simulink subsystem "FMUEngine"  (R2024b)
settings: Solver=VariableStepAuto  StartTime=0.0  StopTime=10.0  RelTol=1e-3
undefined symbols (not defined in the file): Afr, BSFC, CrkAng, EngSpdOut, EngTrq, ExhManGasTemp, FuelFlw, FuelVolFlw, IntkPortFlw, NormAirChrg, PlntEngFuelSg
libraries: autolibhevctrlrcommon x1, autolibpowerinfoutils x1, autolibutils x1
settings Model: ModifiedByFormat=The MathWorks, Inc.  Creator=The MathWorks, Inc.  LastModifiedBy=The MathWorks, Inc.
settings OptimizationCC: ReuseModelBlockBuffer=off
settings DebuggingCC: SubsystemReferenceDiagnosticForUnitTest=warning
settings RTWCC: GPUComputeCapability=3.5

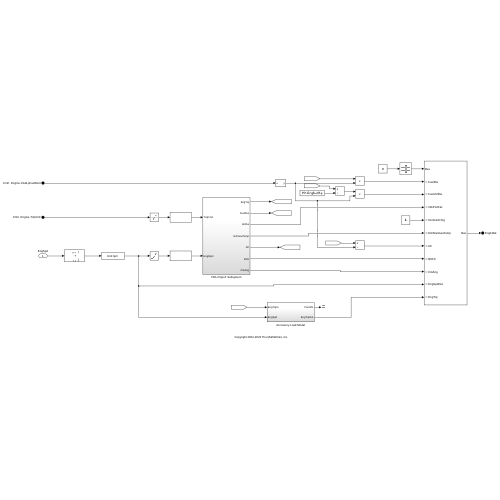
[thumbnail: Simulink's stored preview of the top-level diagram]
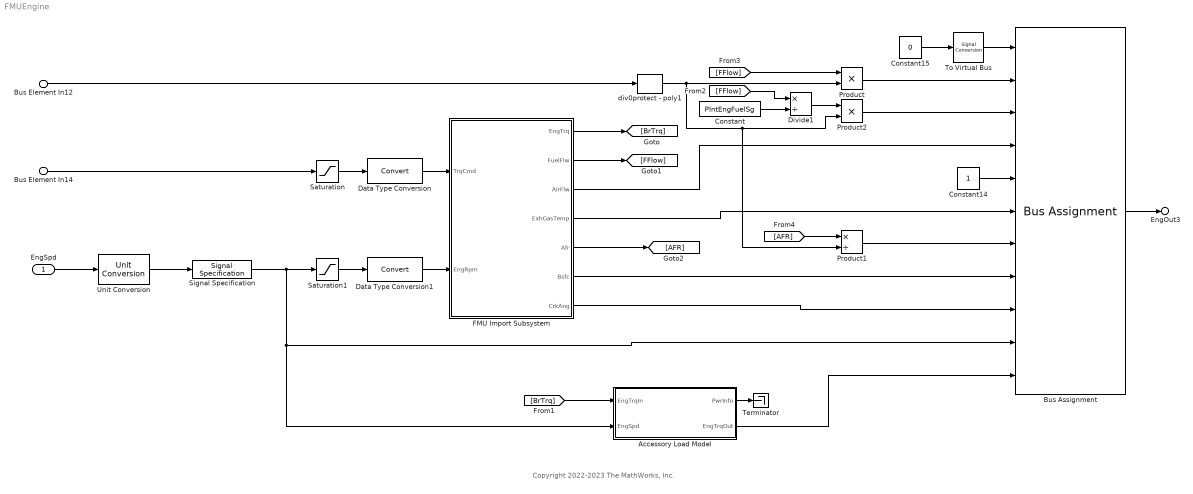
== system FMUEngine ==
  note: Copyright 2022-2023 The MathWorks, Inc.
  EngSpd : Inport  Unit=rad/sec
  Bus Element In12 : Inport  Port=2  PortName=Cntrl  Element=Engine.ClsdLpFuelMult
  Bus Element In14 : Inport  Port=2  PortName=Cntrl  Element=Engine.TrqCmd
  Accessory Load Model : Subsystem
  Bus Assignment : BusAssignment  AssignedSignals=FuelFlw,FuelVolFlw,IntkPortFlw,NormAirChrg,ExhManGasTemp,Afr,BSFC,CrkAng,EngSpdOut,EngTrq
  Constant : Constant  Value=PlntEngFuelSg  SampleTime=-1
  Constant14 : Constant  SampleTime=-1
  Constant15 : Constant  Value=0  OutDataTypeStr=Bus: EngineBUS  SampleTime=Inf
  Data Type Conversion : DataTypeConversion  SaturateOnIntegerOverflow=off  RndMeth=Floor
  Data Type Conversion1 : DataTypeConversion  SaturateOnIntegerOverflow=off  RndMeth=Floor
  Divide1 : Product  Inputs=*/
  FMU Import Subsystem : Subsystem
  Product : Product
  Product1 : Product  Inputs=*/
  Product2 : Product
  Saturation : Saturate  UpperLimit=inf  LowerLimit=0  ZeroCross=off
  Saturation1 : Saturate  UpperLimit=inf  LowerLimit=0  ZeroCross=off
  Signal Specification : SignalSpecification  Unit=rpm
  Terminator : Terminator
  To Virtual Bus : SignalConversion  ConversionOutput=Virtual bus  OverrideOpt=off
  Unit Conversion : UnitConversion
  div0protect - poly1 : autolibutils/div0protect - poly  thresh=0.01  ZeroCross1=off  aMode=aMode
  EngOut3 : Outport  PortName=EngFdbk
  wires:
  Signal Specification/1 -> Saturation1/1, Bus Assignment/10, Accessory Load Model/2(EngSpd)
  [AFR] -> Product1/1
  Constant14/1 -> Bus Assignment/5
  Divide1/1 -> Product2/1
  [FFlow] -> Product/1
  [FFlow] -> Divide1/1
  Constant/1 -> Divide1/2
  [BrTrq] -> Accessory Load Model/1(EngTrqIn)
  Product/1 -> Bus Assignment/2
  EngSpd/1 -> Unit Conversion/1
  Accessory Load Model/2(EngTrqOut) -> Bus Assignment/11
  Bus Element In14/1 -> Saturation/1
  Unit Conversion/1 -> Signal Specification/1
  Bus Element In12/1 -> div0protect - poly1/1
  div0protect - poly1/1 -> Product1/2, Product2/2, Product/2
  Product2/1 -> Bus Assignment/3
  Product1/1 -> Bus Assignment/7
  Accessory Load Model/1(PwrInfo) -> Terminator/1
  Saturation1/1 -> Data Type Conversion1/1
  FMU Import Subsystem/1(EngTrq) -> [BrTrq]
  FMU Import Subsystem/2(FuelFlw) -> [FFlow]
  FMU Import Subsystem/3(AirFlw) -> Bus Assignment/4
  FMU Import Subsystem/4(ExhGasTemp) -> Bus Assignment/6
  FMU Import Subsystem/5(Afr) -> [AFR]
  FMU Import Subsystem/6(Bsfc) -> Bus Assignment/8
  FMU Import Subsystem/7(CrkAng) -> Bus Assignment/9
  Saturation/1 -> Data Type Conversion/1
  Data Type Conversion/1 -> FMU Import Subsystem/1(TrqCmd)
  Data Type Conversion1/1 -> FMU Import Subsystem/2(EngRpm)
  To Virtual Bus/1 -> Bus Assignment/1
  Constant15/1 -> To Virtual Bus/1
  Bus Assignment/1 -> EngOut3/1

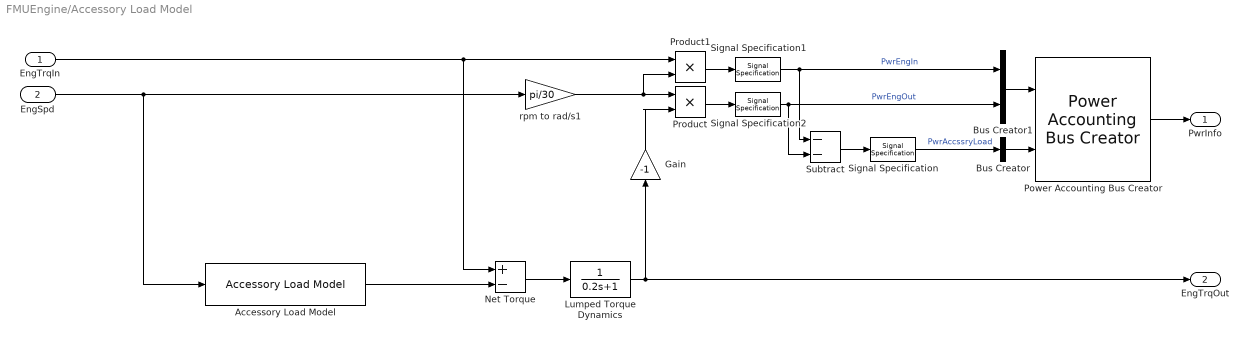
== system FMUEngine/Accessory Load Model ==
  EngTrqIn : Inport
  EngSpd : Inport  Port=2
  Accessory Load Model : autolibhevctrlrcommon/Accessory Load Model  AccPwrTbl=PlntEngAccPwrTbl  AccSpdBpts=PlntEngAccSpdBpt
  Bus Creator : BusCreator  Inputs=1
  Bus Creator1 : BusCreator  Inputs=2
  Gain : Gain  Gain=-1
  Lumped Torque Dynamics : TransferFcn  Denominator=[0.2 1]
  Net Torque : Sum  Inputs=+-
  Power Accounting Bus Creator : autolibpowerinfoutils/Power Accounting Bus Creator  AssctBlkSelPopup=Parent  RefBlkName='libraryname/blkname'  PwrTrnsfrdCheckBox=on  PwrNotTrnsfrdCheckBox=on  PwrStoredCheckBox=off  aMode=6
  Product : Product
  Product1 : Product
  Signal Specification : SignalSpecification  Unit=W
  Signal Specification1 : SignalSpecification  Unit=W
  Signal Specification2 : SignalSpecification  Unit=W
  Subtract : Sum  Inputs=--
  rpm to rad/s1 : Gain  Gain=pi/30
  PwrInfo : Outport  VectorParamsAs1DForOutWhenUnconnected=off
  EngTrqOut : Outport  Port=2  Unit=N*m  VectorParamsAs1DForOutWhenUnconnected=off
  wires:
  Gain/1 -> Product/2
  Signal Specification2/1 -> Bus Creator1/2, Subtract/2  "PwrEngOut"
  Signal Specification1/1 -> Bus Creator1/1, Subtract/1  "PwrEngIn"
  rpm to rad/s1/1 -> Product/1, Product1/2
  Product1/1 -> Signal Specification1/1
  Product/1 -> Signal Specification2/1
  Power Accounting Bus Creator/1 -> PwrInfo/1
  Signal Specification/1 -> Bus Creator/1  "PwrAccssryLoad"
  Subtract/1 -> Signal Specification/1
  EngTrqIn/1 -> Net Torque/1, Product1/1
  Bus Creator1/1 -> Power Accounting Bus Creator/1
  Bus Creator/1 -> Power Accounting Bus Creator/2
  Net Torque/1 -> Lumped Torque Dynamics/1
  Lumped Torque Dynamics/1 -> Gain/1, EngTrqOut/1
  EngSpd/1 -> rpm to rad/s1/1, Accessory Load Model/1
  Accessory Load Model/1 -> Net Torque/2

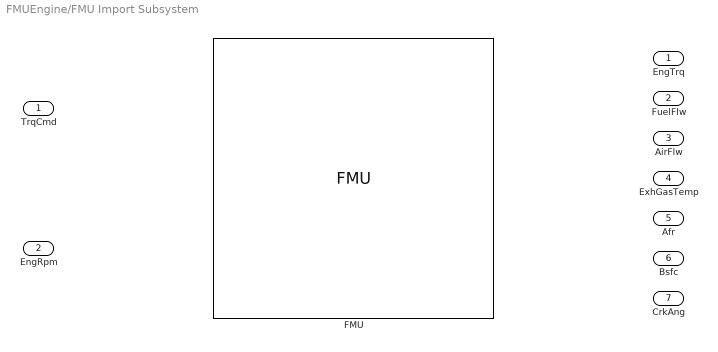
== system FMUEngine/FMU Import Subsystem ==
  TrqCmd : Inport  Description=Commanded brake torque  Unit=N*m
  EngRpm : Inport  Description=Engine speed in rpm  Port=2  Unit=rpm
  FMU : FMU
  EngTrq : Outport  Description=Brake torque  Unit=N*m
  FuelFlw : Outport  Description=Fuel mass flow rate  Port=2  Unit=kg/s
  AirFlw : Outport  Description=Air mass flow rate  Port=3  Unit=kg/s
  ExhGasTemp : Outport  Description=Exhaust gas temperature  Port=4  Unit=K
  Afr : Outport  Description=Air fuel ratio  Port=5  Unit=1
  Bsfc : Outport  Description=Brake specific fuel consumption  Port=6  Unit=g/kW/h
  CrkAng : Outport  Description=Crank angle  Port=7  Unit=deg
